simulink model "eVTOL_Small_nonandlin_algorithm_validation"  (R2024b)
settings: Solver=ode3  StartTime=0.0  StopTime=220  FixedStep=0.02  RelTol=1e-3
undefined symbols (not defined in the file): a_, b, c, c1_, deg, dttrim0, F, g, g1, h1, l1, m, MIL, PARAR, rad, rho, s, T, u_dim, ut, x_dim, xf, xmset, y_dim, yf, ymset, zf, zmset
libraries: simulink x34, aerolibconvert2 x5, aerolibwind2 x2, shared6dof x1
(part 1 of 7)
settings Model: Creator=Septemnicole  LastModifiedBy=23299
settings SolverCC: AlgebraicLoopSolver=TrustRegion
settings DataIOCC: SaveFormat=StructureWithTime  InspectSignalLogs=on  ReturnWorkspaceOutputs=off
settings OptimizationCC: LifeSpan=inf
settings DebuggingCC: UnconnectedInputMsg=warning  UnconnectedOutputMsg=warning  UnconnectedLineMsg=warning  SFExecutionAtInitializationDiag=none  UnderSpecifiedDimensionMsg=warning  ArithmeticOperatorsInVariantConditions=warning
settings HardwareCC: ProdBitPerSizeT=32  ProdBitPerPtrDiffT=32  ProdWordSize=32  ProdHWDeviceType=Specified
settings ModelReferenceCC: EnableRefExpFcnMdlSchedulingChecks=on
settings SFSimCC: SimUseLocalCustomCode=off  CustomCodeUndefinedFunction=UseInterfaceOnly
settings RTWCC: RTWUseLocalCustomCode=off  GPUComputeCapability=3.5
settings CodeAppCC: StateflowObjectComments=on

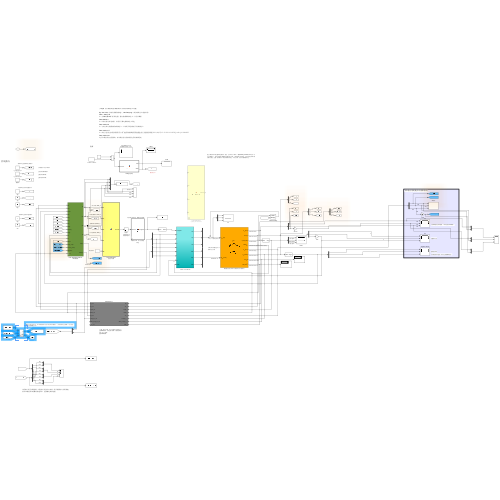
[thumbnail: Simulink's stored preview of the top-level diagram]
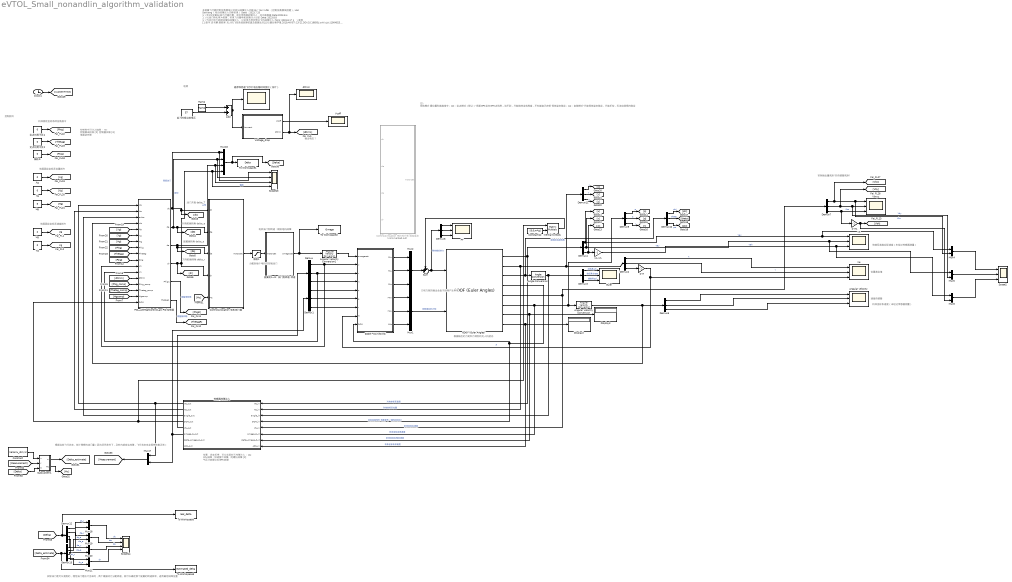
== system eVTOL_Small_nonandlin_algorithm_validation ==
  note: 实际油门是可以测到的，理性油门是估计出来的，两个根据动力分配转速，就可以确定那个旋翼的转速异常，进而确定故障位置
  note: 根据当前飞行状态，估计理想的油门量（因为闭环条件下，及时内部发生故障，飞行状态也会很快恢复正常）
  note: 方向舵偏转角 delta_r
  note: 副翼偏转角 delta_a
  note: 升降舵偏转角 delta_e
  note: 油门开度 delta_T
  note: 电机油门到转速：模拟电机故障
  note: 机体固定坐标系欧拉角指令
  note: 实际输出量观测(非传感器观测)
  note: 位置、姿态反馈，可以实现如下故障注入：
      | [1] IMU故障：加速度计故障、陀螺仪故障
      | [2] 气压计故障
      | [3] GPS故障
  note: 输出电压？
  note: 分配到每个电机的控制油门
  note: 多旋翼飞行器控制仿真模块以及部分故障注入功能
      |
      | By: Yan Xufei（控制仿真模块搭建）, Han Danyang（部分故障注入功能实现）
      | Date：2023.7.20
      | 1）完成8旋翼16轴飞行器位置、姿态传感器故障注入，并记录数据
      |
      | Date:2023.8.4
      | 1）以油门转化率为依据，实现飞行器电机故障注入设定
      |
      | Date: 2023.8.8
      | 1）气动力和力矩模块增加故障注入，以实现不受控情况下的故障注入
      |
      | Date: 2023.8.17
      | 1）参考 [1]彭宇,史书慧,郭凯等.无人机飞控系统故障仿真及数据生成[J].仪器仪表学报,2019,40(07):13-21.DOI:10.19650/j.cnki.cjsi.J1904825.
      |
      | Date: 2023.9.21
      | 1) 引入线性状态方程模块，对比线性化与复杂模型之间的相似程度
  note: 控制指令可注入故障：
      |
      | [1] 控制器未校准
      |
      | [2] 控制器失联
      |
      | [3] 地面站失联
  note: [1]: 导航模式-跟位置和速度指令；[2]：定点模式（默认）-根据GPS定在GPS点和高度（气压计+RTK）；[3]:定高模式-GPS水平模式读不到，只能维持当前高度，不知道自己在哪-保持姿态稳定；[4]：自稳模式-只能保持姿态稳定，只能手控，无法自我保持稳定
  note: 力和力矩的输出会由于故障产生异常
  note: 地轴系速度实际速度（未经过传感器测量）
  note: 根据输出的力矩和力得到的无人机姿态
  note: 电源
  note: 控制指令
  note: 位置真实值
  note: 速度传感器
  note: 地面固定坐标系位置指令
  note: 地面固定坐标系速度指令
  note: 机体坐标系速度（未经过传感器测量）
  " Angular velocity" : Scope  NumInputPorts=3
  6DOF (Euler Angles) : shared6dof/6DOF (Euler Angles)  units=Metric (MKS)  mtype=Fixed  rep=Euler Angles  xme_0=[0 0 0]  Vm_0=[0 0 0]  eul_0=[0/57.3 0/57.3 0/57.3]  pm_0=[0 0 0]  mass_0=Mass  mass_e=0.5  mass_f=2.0  inertia=Inertia  inertia_e=eye(3)  inertia_f=2*eye(3)  k_quat=1.0  vre_flag=on  abi_flag=off  aMode=aMode  xme_statename=''  Vm_statename=''  eul_statename=''  quat_statename=''  pm_statename=''  mass_statename=''
  Add : Sum
  Angle Conversion : aerolibconvert2/Angle Conversion  IU=rad  OU=deg
  Angular Velocity Conversion : aerolibconvert2/Angular Velocity Conversion  IU=rad/s  OU=deg/s
  Angular Velocity Conversion1 : aerolibconvert2/Angular Velocity Conversion  IU=rpm  OU=rad/s
  Clock1 : Clock
  Constant : Constant  Value=zeros(u_dim,1)
  Constant12 : Constant  Value=[0,0,m*g]
  ControlAllocation 电机执行器 : MATLAB Function  TreatAsAtomicUnit=on
  ControlAllocation 电机执行器-原始版本 : MATLAB Function  Commented=on  TreatAsAtomicUnit=on
  Demux{,1..7,9..11} (11 alike) : Demux  Outputs=3
  Demux12 : Demux
  Demux13 : Demux
  Display2 : Display
  Display3 : Display
  Euler : Scope  NumInputPorts=3
  FT : Scope  NumInputPorts=3
  Hg : Constant  Value=5
  Inertial to Body : Product  Multiplication=Matrix(*)  InputSameDT=on  SaturateOnIntegerOverflow=on  OutDataTypeStr=Inherit: Same as first input
  Mux1 : Mux  Inputs=3
  Mux16 : Mux
  Mux{4..6,17..21} (8 alike) : Mux  Inputs=2
  Mux2 : Mux  Inputs=3
  PID—AttHighControlLaw PID控制器 : Subsystem  mask{Ea=1}
      mask prompts: Ea "Euler angle control enable(1=disable, 2=enable)"
  Ramp : simulink/Sources/Ramp  slope=-0.05  start=0  InitialOutput=0
  Scope13 : Scope  NumInputPorts=4
  Scope14 : Scope  NumInputPorts=4
  Scope2 : Scope  NumInputPorts=3
  Subsystem1 : Subsystem
  Sum : Sum  Inputs=++|
  To Workspace : ToWorkspace  VariableName=real_delta  SaveFormat=Timeseries  SampleTime=-1
  To Workspace1 : ToWorkspace  VariableName=Delta  SaveFormat=Timeseries  SampleTime=-1
  To Workspace2 : ToWorkspace  VariableName=Omega  SaveFormat=Timeseries  SampleTime=-1
  To Workspace3 : ToWorkspace  VariableName=estimated_delta  SaveFormat=Timeseries  SampleTime=-1
  Ug : Constant  Value=2
  Vbxyz : Scope  NumInputPorts=3
  Vcoff : Scope
  Ve : Scope  NumInputPorts=3
  Vg : Constant  Value=0
  Voltage_drop : MATLAB Function  TreatAsAtomicUnit=on
  Vz-Vh : Gain  Gain=-1
  Xe : Scope  NumInputPorts=3
  Xg : Constant  Value=0
  Yg : Constant  Value=0
  Z-H : Gain  Gain=-1
  Z-H1 : Gain  Gain=-1
  dttrim : Scope
  传感器故障注入 : Subsystem  mask{Pmn=0}
      mask prompts: Pmn "the power of meansurement noise (E[S_xx]=(theta^2)/2F)"
  偏航G : Constant  Value=0
  各部件气动力和力矩 : Subsystem
  定点时用不到1 : Constant  Value=0
  定点时用不到2 : Constant  Value=0
  悬停和低速飞行时 电压随时间变化（估计） : Scope
  旋翼组1~8：油门到转速 转速 : MATLAB Function  TreatAsAtomicUnit=on  mask{L_r=1}
      mask prompts: L_r "Power loss rate from motor to omega"
  起飞时候当前电压 : Constant  Value=57
  限幅1 : Saturate  UpperLimit=1  LowerLimit=0.1
  tag scope: Ug=global, Vg=global
  wires:
  Inertial to Body/1 -> Sum/1
  6DOF (Euler Angles)/7 -> 传感器故障注入/7(delta_omega_b_in), Display3/1  "机体坐标系角加速度"
  Constant12/1 -> Inertial to Body/2
  Demux1/2 -> 各部件气动力和力矩/6(q)
  Demux1/1 -> 各部件气动力和力矩/5(p)
  Demux1/3 -> 各部件气动力和力矩/7(r)
  6DOF (Euler Angles)/8 -> 传感器故障注入/8(Abb_in), Display2/1  "机体坐标系加速度"
  6DOF (Euler Angles)/6 -> Demux9/1, Angular Velocity Conversion/1, 传感器故障注入/6(omega_b_in)  "机体坐标系角速度"
  Mux2/1 -> Sum/2
  6DOF (Euler Angles)/3 -> Demux10/1, Angle Conversion/1  "固有欧拉旋转角"
  Demux/3 -> 各部件气动力和力矩/4(w)
  [Thetag] -> PID—AttHighControlLaw PID控制器/9(Thetag)
  [Phig] -> PID—AttHighControlLaw PID控制器/8(Phig)
  Demux2/2 -> Xe/2  "Y"
  Demux2/1 -> Xe/1  "X"
  Demux2/3 -> Z-H/1
  Demux3/1 -> Euler/1  "滚转角phi"
  Demux3/2 -> Euler/2  "俯仰角theta"
  Demux3/3 -> Euler/3  "偏航角psi"
  Demux4/1 -> [u], Ve/1, Mux4/1  "Vex"
  Demux4/2 -> [v], Mux5/1, Ve/2  "Vey"
  Demux4/3 -> [w], Vz-Vh/1
  Demux5/2 -> " Angular velocity"/2
  Demux5/1 -> " Angular velocity"/1
  Demux5/3 -> " Angular velocity"/3
  Add/1 -> 悬停和低速飞行时 电压随时间变化（估计）/1, Voltage_drop/1(Vcurrent)
  起飞时候当前电压/1 -> Add/2
  Voltage_drop/2(dttrim) -> [dttrim], dttrim/1
  Voltage_drop/1(Vcoff) -> Vcoff/1
  Ramp/1 -> Add/1
  Demux6/3 -> FT/3
  Demux6/2 -> FT/2
  Demux6/1 -> FT/1
  Mux1/1 -> 6DOF (Euler Angles)/2  "刚体施加的力矩"
  Sum/1 -> 6DOF (Euler Angles)/1, Demux6/1  "刚体施加的力"
  各部件气动力和力矩/1(FAx) -> Mux2/1
  各部件气动力和力矩/2(FAy) -> Mux2/2
  各部件气动力和力矩/3(FAz) -> Mux2/3
  各部件气动力和力矩/4(MAx) -> Mux1/1
  各部件气动力和力矩/5(MAy) -> Mux1/2
  各部件气动力和力矩/6(MAz) -> Mux1/3
  Vz-Vh/1 -> Mux6/1, Ve/3  "Veh"
  [dttrim] -> PID—AttHighControlLaw PID控制器/13(dttrim)
  Angular Velocity Conversion1/1 -> 各部件气动力和力矩/1(omegaset)
  ControlAllocation 电机执行器/1(motorset) -> 限幅1/1
  Demux/2 -> 各部件气动力和力矩/3(v), PID—AttHighControlLaw PID控制器/12(v1)
  Demux/1 -> PID—AttHighControlLaw PID控制器/11(u1), 各部件气动力和力矩/2(u)
  Z-H/1 -> 各部件气动力和力矩/8(H), Xe/3  "H"
  [Xg] -> PID—AttHighControlLaw PID控制器/5(Xg)
  [Yg] -> PID—AttHighControlLaw PID控制器/6(Yg)
  Angular Velocity Conversion/1 -> Demux5/1, PID—AttHighControlLaw PID控制器/4(wb)
  Demux7/1 -> [Vbx], Mux4/2, Vbxyz/1  "Vbx"
  Demux7/2 -> Mux5/2, Vbxyz/2, [Vby]  "Vby"
  6DOF (Euler Angles)/5 -> Demux7/1, 传感器故障注入/5(Vb_in)  "机体坐标系速度"
  PID—AttHighControlLaw PID控制器/5(Phig1) -> [PhigR]  "期望滚转角"
  PID—AttHighControlLaw PID控制器/6(thetag1) -> [ThetagR]  "期望俯仰角"
  [Hg] -> PID—AttHighControlLaw PID控制器/7(Hg)
  [Phig_comp] -> PID—AttHighControlLaw PID控制器/14(Phig_comp)
  [Thetag_comp] -> PID—AttHighControlLaw PID控制器/15(Thetag_comp)
  偏航G/1 -> [Psig]
  [Psig] -> PID—AttHighControlLaw PID控制器/10(Psig)
  Xg/1 -> [Xg]
  Hg/1 -> [Hg]
  定点时用不到1/1 -> [Phig]
  定点时用不到2/1 -> [Thetag]
  [Hgcomp] -> PID—AttHighControlLaw PID控制器/16(Hgcomp)
  Z-H1/1 -> Mux6/2, [Vbh]
  Demux7/3 -> Z-H1/1, Vbxyz/3  "Vbz"
  限幅1/1 -> 旋翼组1~8：油门到转速 转速/1(motorset)
  PID—AttHighControlLaw PID控制器/1(dt) -> Scope13/1, Mux16/1, [dt], ControlAllocation 电机执行器/1(dt)  "高度油门"
  PID—AttHighControlLaw PID控制器/2(de) -> [de], ControlAllocation 电机执行器/2(de), Scope13/2, Mux16/2  "俯仰"
  PID—AttHighControlLaw PID控制器/3(da) -> ControlAllocation 电机执行器/3(da), [da], Scope13/3, Mux16/3  "滚转"
  PID—AttHighControlLaw PID控制器/4(dr) -> [dr], ControlAllocation 电机执行器/4(dr), Scope13/4, Mux16/4  "偏航"
  6DOF (Euler Angles)/1 -> Demux4/1, 传感器故障注入/1(Ve_in)  "对地坐标系速度"
  传感器故障注入/1(Ve_out) -> Mux17/1, PID—AttHighControlLaw PID控制器/1(Ve)
  传感器故障注入/2(Xe_out) -> PID—AttHighControlLaw PID控制器/2(Xe)
  6DOF (Euler Angles)/2 -> Demux2/1, Demux11/1, 传感器故障注入/2(Xe_in)  "对地坐标系位置"
  Angle Conversion/1 -> 传感器故障注入/3(angle_in), Demux3/1
  传感器故障注入/3(angle_out) -> PID—AttHighControlLaw PID控制器/3(euler)
  6DOF (Euler Angles)/4 -> 传感器故障注入/4(DCM_in), 各部件气动力和力矩/9(DCM)  "坐标变换矩阵(地面参考->固有坐标系)"
  传感器故障注入/5(Vb_out) -> Demux/1
  传感器故障注入/6(omega_b_out) -> Demux1/1, Mux17/2
  传感器故障注入/4(DCM_out) -> Inertial to Body/1, PID—AttHighControlLaw PID控制器/17(DCM)
  Yg/1 -> [Yg]
  Vg/1 -> [Vg]
  Ug/1 -> [Ug]
  旋翼组1~8：油门到转速 转速/1(omegaset) -> Angular Velocity Conversion1/1, To Workspace2/1
  Mux4/1 -> Scope2/1
  Mux5/1 -> Scope2/2
  Mux6/1 -> Scope2/3
  Demux9/1 -> [p]  "p"
  Demux9/2 -> [q]  "q"
  Demux9/3 -> [r]  "r"
  Demux10/1 -> [phi]  "phi"
  Demux10/2 -> [theta]  "theta"
  Demux10/3 -> [psi]  "psi"
  Demux11/1 -> [x]  "x"
  Demux11/2 -> [y]  "y"
  Demux11/3 -> [z]  "z"
  Clock1/1 -> [systemTime]
  Mux16/1 -> [Delta], To Workspace1/1
  [Mc] -> ControlAllocation 电机执行器/5(Mc)
  Mux17/1 -> [Measurement]
  [Measurement] -> Subsystem1/2(y)
  Subsystem1/1(w) -> [Delta_estimate]
  Subsystem1/2(Mc) -> [Mc]
  [Delta_estimate] -> To Workspace3/1, Demux13/1
  [Delta] -> To Workspace/1, Demux12/1
  Demux12/1 -> Mux18/1  "dt_r"
  Demux13/1 -> Mux18/2  "dt_e"
  Demux12/2 -> Mux19/1  "de_r"
  Demux13/2 -> Mux19/2  "de_e"
  Demux12/3 -> Mux20/1  "da_r"
  Demux13/3 -> Mux20/2  "da_e"
  Demux12/4 -> Mux21/1  "dr_r"
  Demux13/4 -> Mux21/2  "dr_e"
  Mux18/1 -> Scope14/1  "dt"
  Mux19/1 -> Scope14/2  "de"
  Mux20/1 -> Scope14/3  "da"
  Mux21/1 -> Scope14/4  "dr"
  [Delta] -> Subsystem1/3(ww)
  Constant/1 -> Subsystem1/1(u)

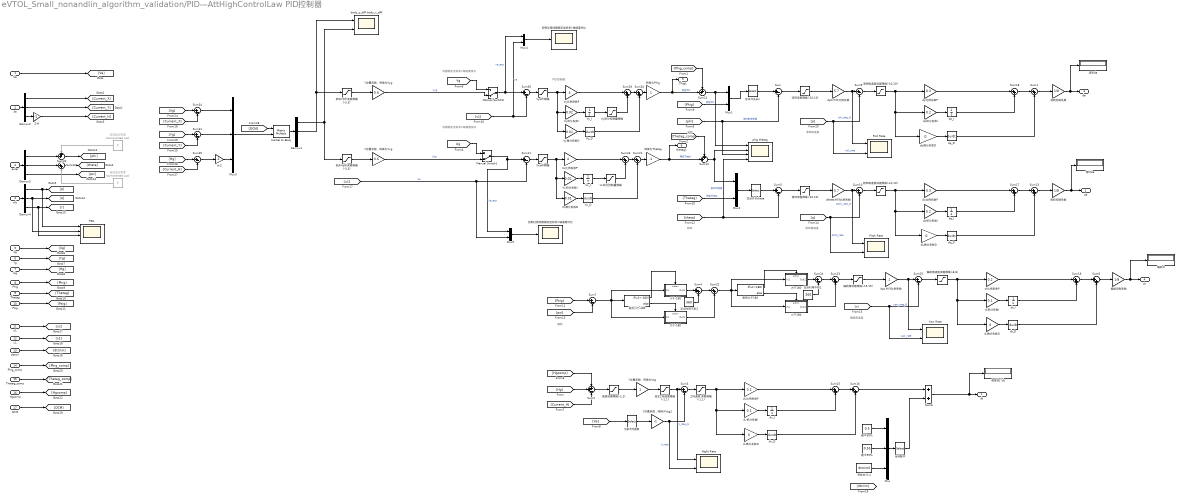
== system eVTOL_Small_nonandlin_algorithm_validation/PID—AttHighControlLaw PID控制器 ==
  note: 地面固定坐标系X轴速度指令
  note: 地面固定坐标系Y轴速度指令
  note: PID控制器
  note: 偏航
  note: 滚转角速度
  note: 俯仰角速度
  note: 俯仰
  note: 滚转
  note: 偏航角速度
  Ve : Inport
  Xe : Inport  Port=2
  euler : Inport  Port=3
  wb : Inport  Port=4
  Xg : Inport  Port=5
  Yg : Inport  Port=6
  Hg : Inport  Port=7
  Phig : Inport  Port=8
  Thetag : Inport  Port=9
  Psig : Inport  Port=10
  u1 : Inport  Port=11
  v1 : Inport  Port=12
  dttrim : Inport  Port=13
  Phig_comp : Inport  Port=14
  Thetag_comp : Inport  Port=15
  Hgcomp : Inport  Port=16
  DCM : Inport  Port=17
  Demux{1..4} (4 alike) : Demux  Outputs=3
  H-Z : Gain  Gain=-1
  Hight Rate : Scope  NumInputPorts=2
  Inertial to Body : Product  Multiplication=Matrix(*)  InputSameDT=on  SaturateOnIntegerOverflow=on  OutDataTypeStr=Inherit: Same as first input
  Manual Switch1 : ManualSwitch  CurrentSetting=0
  Manual Switch8 : ManualSwitch  CurrentSetting=0
  Mux : Mux  Inputs=3
  Mux{1..2,4..5} (4 alike) : Mux  Inputs=2
  Mux3 : Mux  Inputs=3
  PSI1 : Scope  NumInputPorts=4
  Pitch Rate : Scope  NumInputPorts=2
  Roll Rate : Scope  NumInputPorts=2
  Sum{,3,5,7,9..11,24..25,30..31,34..35} (13 alike) : Sum  Inputs=|+-
  Sum{1,4,8,13,15..23,26,29,33} (16 alike) : Sum  Inputs=|++
  Sum12 : Sum  Inputs=++|
  Sum14 : Sum  Inputs=++|
  Sum2 : Sum  Inputs=++-
  Sum32 : Sum  Inputs=++|
  Sum6 : Sum
  Vx_D : Derivative
  Vx_I : Integrator
  Vxdiff限幅 : Saturate  UpperLimit=2.4  LowerLimit=-2.4
  Vx微分系数D : Gain  Gain=0.01
  Vx比例系数P : Gain  Gain=4
  Vx积分控制量限幅 : Saturate  UpperLimit=2  LowerLimit=-2
  Vx积分系数I : Gain  Gain=0.02
  Vy_D : Derivative
  Vy_I : Integrator
  Vydiff限幅 : Saturate  UpperLimit=2.4  LowerLimit=-2.4
  Vy微分系数D : Gain  Gain=0.01
  Vy比例系数P : Gain  Gain=4
  Vy积分控制量限幅 : Saturate  UpperLimit=2  LowerLimit=-2
  Vy积分系数I : Gain  Gain=0.02
  X位置系数，转换为Vxg : Gain  Gain=0.6
  Yaw Rate : Scope  NumInputPorts=2
  Y位置系数，转换为Vyg : Gain  Gain=0.6
  Y位置系数，转换为Vzg : Gain
  Y位置系数，转换为Vzg1 : Gain  Gain=-1
  Z-H : Gain  Gain=-1
  Z向速度 误差限幅 (-1,1) : Saturate  UpperLimit=1  LowerLimit=-1
  body_y_diff body_x_diff : Scope  NumInputPorts=2
  dp_D : Derivative
  dp_I : Integrator
  dphi外环比例系数 : Gain  Gain=5.7
  dpsi外环比例系数 : Gain
  dp微分系数D : Gain  Gain=0
  dp比例系数P : Gain  Gain=0.3
  dp积分系数I : Gain  Gain=0.2
  dq_D : Derivative
  dq_I : Integrator
  dq微分系数D : Gain  Gain=0
  dq比例系数P : Gain  Gain=0.3
  dq积分系数I : Gain  Gain=0.2
  dr_D : Derivative
  dr_I : Integrator
  dr微分系数D : Gain  Gain=0
  dr比例系数P : Gain  Gain=0.2
  dr积分系数I : Gain  Gain=0.1
  dtheta外环比例系数 : Gain  Gain=5.7
  dv_D : Derivative
  dv_I : Integrator
  dv微分系数D : Gain  Gain=0
  dv比例系数P : Gain  Gain=0.2
  dv积分系数I : Gain  Gain=0.1
  phig thetag : Scope  NumInputPorts=4
  俯仰de : Display
  俯仰姿态零漂 : Constant  Commented=on  Value=0
  俯仰控制系数 : Gain  Gain=1/8
  俯仰角速度误差限幅(-10,10) : Saturate  UpperLimit=10  LowerLimit=-10
  "俯仰误差限幅(-10,10) " : Saturate  UpperLimit=10  LowerLimit=-10
  偏航dr : Display
  偏航控制系数 : Gain  Gain=1/8
  "偏航角误差限幅(-15,15) " : Saturate  UpperLimit=15  LowerLimit=-15
  偏航角速度误差限幅(-8,8) : Saturate  UpperLimit=8  LowerLimit=-8
  "初始dt 0.4 " : Constant  Value=dttrim0
  大于-180 : Subsystem  TreatAsAtomicUnit=on
  大于180 : Subsystem  TreatAsAtomicUnit=on
  定点开关phi : Selector  InputPortWidth=2  IndexOptions=Index vector (dialog)  Indices=[Ea]  OutputSizes=1
  定点开关theta : Selector  InputPortWidth=2  IndexOptions=Index vector (dialog)  Indices=[Ea]  OutputSizes=1
  定点时用不到1 : Constant  Value=360
  定点时用不到2 : Constant  Value=360
  小于-180 : Subsystem  TreatAsAtomicUnit=on
  小于180 : Subsystem  TreatAsAtomicUnit=on
  当前Z向速度 : Selector  InputPortWidth=3  IndexOptions=Index vector (dialog)  Indices=[3]  OutputSizes=1
  当前配平 : Selector  InputPortWidth=3  IndexOptions=Index vector (dialog)  Indices=[3]  OutputSizes=1
  控制过程地面固定坐标系X轴速度对比 : Scope
  控制过程地面固定坐标系Y轴速度对比 : Scope
  是否大于180 : If  IfExpression=u1>180
  是否小于-180 : If  IfExpression=u1<-180
  机体Xdiff误差限幅 (-3,3) : Saturate  UpperLimit=3  LowerLimit=-3
  机体Ydiff误差限幅 (-3,3) : Saturate  UpperLimit=3  LowerLimit=-3
  滚转da : Display
  滚转姿态零漂 : Constant  Commented=on  Value=0
  滚转控制系数 : Gain  Gain=1/8
  滚转角速度误差限幅(-10,10) : Saturate  UpperLimit=10  LowerLimit=-10
  "滚转误差限幅(-10,10) " : Saturate  UpperLimit=10  LowerLimit=-10
  给定Z向速度限幅 (-1,1) : Saturate  UpperLimit=1  LowerLimit=-1
  转换为Phig : Gain
  转换为Thetag : Gain  Gain=-1
  "配平50% " : Constant  Value=0.5
  配平55% : Constant  Value=0.55
  高度油门dt : Display
  高度误差限幅(-2,2) : Saturate  UpperLimit=2  LowerLimit=-2
  dt : Outport  VectorParamsAs1DForOutWhenUnconnected=off
  de : Outport  Port=2  VectorParamsAs1DForOutWhenUnconnected=off
  da : Outport  Port=3  VectorParamsAs1DForOutWhenUnconnected=off
  dr : Outport  Port=4  VectorParamsAs1DForOutWhenUnconnected=off
  Phig1 : Outport  Port=5  VectorParamsAs1DForOutWhenUnconnected=off
  thetag1 : Outport  Port=6  VectorParamsAs1DForOutWhenUnconnected=off
  wires:
  euler/1 -> Demux3/1
  Demux4/1 -> PSI1/1, [p]
  Demux4/2 -> PSI1/2, [q]
  Thetag/1 -> [Thetag]
  wb/1 -> Demux4/1
  Hg/1 -> [Hg]
  Demux4/3 -> PSI1/3, [r]
  Yg/1 -> [Yg]
  Demux3/3 -> [psi]
  Demux2/3 -> Z-H/1
  Xe/1 -> Demux2/1
  Psig/1 -> [Psig]
  u1/1 -> [u1]
  v1/1 -> [v1]
  dttrim/1 -> [dttrim]
  Sum32/1 -> [phi]
  Demux3/1 -> Sum32/2
  滚转姿态零漂/1 -> Sum32/1
  Sum33/1 -> [theta]
  Demux3/2 -> Sum33/1
  俯仰姿态零漂/1 -> Sum33/2
  Demux2/1 -> [Current_X]
  Demux2/2 -> [Current_Y]
  Z-H/1 -> [Current_H]
  Xg/1 -> [Xg]
  Phig/1 -> [Phig]
  Sum22/1 -> 大于180/1(In1), 小于180/1(In1), 是否大于180/1
  Sum16/1 -> Sum6/1
  Mux2/1 -> 定点开关theta/1
  Sum18/1 -> Sum1/1
  dtheta外环比例系数/1 -> Pitch Rate/1, Sum10/1  "pitch_rate_G"
  Vy积分系数I/1 -> Vy_I/1
  配平55%/1 -> Mux/2
  Y位置系数，转换为Vzg1/1 -> Hight Rate/2, Sum3/2  "h_rate"
  是否小于-180/1 -> 小于-180/Action
  [p] -> Roll Rate/2, Sum9/2  "roll_rate"
  dq积分系数I/1 -> dq_I/1
  Sum20/1 -> 转换为Phig/1
  dp_D/1 -> Sum1/2
  [v1] -> Mux4/2, Sum30/2  "Ve"
  Y位置系数，转换为Vyg/1 -> Manual Switch8/2  "Vyg"
  Vx_I/1 -> Vx积分控制量限幅/1
  Sum21/1 -> 转换为Thetag/1
  dphi外环比例系数/1 -> Roll Rate/1, Sum9/1  "roll_rate_G"
  dq_D/1 -> Sum13/2
  Vx积分系数I/1 -> Vx_I/1
  Sum15/1 -> Sum16/1
  dp_I/1 -> Sum18/2
  dv_I/1 -> Sum15/2
  俯仰角速度误差限幅(-10,10)/1 -> dq微分系数D/1, dq积分系数I/1, dq比例系数P/1
  dq比例系数P/1 -> Sum17/1
  [Ve] -> 当前Z向速度/1
  [theta] -> Sum5/2, phig thetag/4  "俯仰传感器"
  Vy微分系数D/1 -> Vy_D/1
  Vy积分控制量限幅/1 -> Sum29/2
  Vy_I/1 -> Vy积分控制量限幅/1
  俯仰控制系数/1 -> 俯仰de/1, de/1
  "偏航角误差限幅(-15,15) "/1 -> dpsi外环比例系数/1
  Vydiff限幅/1 -> Vy微分系数D/1, Vy积分系数I/1, Vy比例系数P/1
  Sum8/1 -> 偏航控制系数/1
  机体Ydiff误差限幅 (-3,3)/1 -> Y位置系数，转换为Vyg/1
  Vxdiff限幅/1 -> Vx微分系数D/1, Vx积分系数I/1, Vx比例系数P/1
  大于180/1(Out1) -> Sum24/1
  Vx比例系数P/1 -> Sum26/1
  dr_I/1 -> Sum19/2
  Mux1/1 -> 定点开关phi/1
  给定Z向速度限幅 (-1,1)/1 -> Hight Rate/1, Sum3/1  "h_rate_G"
  转换为Thetag/1 -> Sum14/2, thetag1/1  "期望Theta"
  滚转控制系数/1 -> 滚转da/1, da/1
  转换为Phig/1 -> Phig1/1, Sum12/2  "期望Phi"
  dv_D/1 -> Sum16/2
  [q] -> Pitch Rate/2, Sum10/2  "pitch_rate"
  Vy_D/1 -> Sum20/2
  dv微分系数D/1 -> dv_D/1
  dv积分系数I/1 -> dv_I/1
  dr积分系数I/1 -> dr_I/1
  dq微分系数D/1 -> dq_D/1
  Sum13/1 -> 俯仰控制系数/1
  [Psig] -> Sum7/1
  dr微分系数D/1 -> dr_D/1
  偏航角速度误差限幅(-8,8)/1 -> dr微分系数D/1, dr积分系数I/1, dr比例系数P/1
  dq_I/1 -> Sum17/2
  dv比例系数P/1 -> Sum15/1
  Sum17/1 -> Sum13/1
  Sum19/1 -> Sum8/1
  dp积分系数I/1 -> dp_I/1
  偏航控制系数/1 -> 偏航dr/1, dr/1
  Y位置系数，转换为Vzg/1 -> 给定Z向速度限幅 (-1,1)/1
  [psi] -> Sum7/2
  Vx微分系数D/1 -> Vx_D/1
  Sum10/1 -> 俯仰角速度误差限幅(-10,10)/1
  Sum30/1 -> Vydiff限幅/1
  [phi] -> phig thetag/3, Sum/2  "滚转角传感器"
  定点开关phi/1 -> Sum/1
  Vy比例系数P/1 -> Sum29/1
  Vx积分控制量限幅/1 -> Sum26/2
  "初始dt 0.4 "/1 -> Mux/3
  X位置系数，转换为Vxg/1 -> Manual Switch1/2  "Uxg"
  定点时用不到1/1 -> Sum24/2
  [Thetag] -> Mux2/2  "期望Theta"
  机体Xdiff误差限幅 (-3,3)/1 -> X位置系数，转换为Vxg/1
  Sum5/1 -> "俯仰误差限幅(-10,10) "/1
  是否小于-180/2 -> 大于-180/Action
  高度误差限幅(-2,2)/1 -> Y位置系数，转换为Vzg/1
  dpsi外环比例系数/1 -> Yaw Rate/1, Sum25/1  "yaw_rate_G"
  Z向速度 误差限幅 (-1,1)/1 -> dv微分系数D/1, dv积分系数I/1, dv比例系数P/1
  Sum7/1 -> 大于-180/1(In1), 小于-180/1(In1), 是否小于-180/1
  Sum3/1 -> Z向速度 误差限幅 (-1,1)/1
  dp微分系数D/1 -> dp_D/1
  是否大于180/2 -> 小于180/Action
  是否大于180/1 -> 大于180/Action
  dr比例系数P/1 -> Sum19/1
  Mux/1 -> 当前配平/1
  Sum23/1 -> "偏航角误差限幅(-15,15) "/1
  定点开关theta/1 -> Sum5/1
  Sum2/1 -> 高度误差限幅(-2,2)/1
  Sum25/1 -> 偏航角速度误差限幅(-8,8)/1
  [r] -> Yaw Rate/2, Sum25/2  "yaw_rate"
  当前配平/1 -> Sum6/2
  "滚转误差限幅(-10,10) "/1 -> dphi外环比例系数/1
  Sum24/1 -> Sum23/1
  dp比例系数P/1 -> Sum18/1
  Sum4/1 -> Sum22/1
  小于180/1(Out1) -> Sum23/2
  "俯仰误差限幅(-10,10) "/1 -> dtheta外环比例系数/1
  Sum11/1 -> Vxdiff限幅/1
  Sum6/1 -> 高度油门dt/1, dt/1
  定点时用不到2/1 -> Sum4/2
  [Phig] -> Mux1/2  "期望Phi"
  Sum9/1 -> 滚转角速度误差限幅(-10,10)/1
  "配平50% "/1 -> Mux/1
  当前Z向速度/1 -> Y位置系数，转换为Vzg1/1
  滚转角速度误差限幅(-10,10)/1 -> dp比例系数P/1, dp微分系数D/1, dp积分系数I/1
  大于-180/1(Out1) -> Sum22/2
  dr_D/1 -> Sum8/2
  Sum1/1 -> 滚转控制系数/1
  小于-180/1(Out1) -> Sum4/1
  Sum/1 -> "滚转误差限幅(-10,10) "/1
  Phig_comp/1 -> [Phig_comp]
  Thetag_comp/1 -> [Thetag_comp]
  Sum12/1 -> phig thetag/1, Mux1/1
  [Phig_comp] -> Sum12/1
  Sum29/1 -> Sum20/1
  [Thetag_comp] -> Sum14/1
  Sum26/1 -> Sum21/1
  Vx_D/1 -> Sum21/2
  Sum14/1 -> Mux2/1, phig thetag/2
  [Hg] -> Sum2/2
  [Current_H] -> Sum2/3
  Demux1/1 -> 机体Xdiff误差限幅 (-3,3)/1, body_y_diff body_x_diff/2
  Demux1/2 -> body_y_diff body_x_diff/1, 机体Ydiff误差限幅 (-3,3)/1
  Sum34/1 -> Mux3/1
  [Hg] -> Sum35/1
  Inertial to Body/1 -> Demux1/1
  Mux3/1 -> Inertial to Body/2
  [Current_X] -> Sum34/2
  [Xg] -> Sum34/1
  [Current_Y] -> Sum31/2
  [Yg] -> Sum31/1
  H-Z/1 -> Mux3/3
  [Current_H] -> Sum35/2
  Sum35/1 -> H-Z/1
  Sum31/1 -> Mux3/2
  [DCM] -> Inertial to Body/1
  DCM/1 -> [DCM]
  Hgcomp/1 -> [Hgcomp]
  [Hgcomp] -> Sum2/1
  Ve/1 -> [Ve]
  [Vg] -> Manual Switch8/1
  [Ug] -> Manual Switch1/1
  Manual Switch8/1 -> Mux4/1, Sum30/1  "Ve_exp"
  Mux4/1 -> 控制过程地面固定坐标系Y轴速度对比/1
  [u1] -> Mux5/2, Sum11/2  "Ve"
  Mux5/1 -> 控制过程地面固定坐标系X轴速度对比/1
  Manual Switch1/1 -> Mux5/1, Sum11/1  "Ue_exp"

== system eVTOL_Small_nonandlin_algorithm_validation/Subsystem1 ==
  note: 实测油门总量
  note: 估计油门总量
  u : Inport
  y : Inport  Port=2
  ww : Inport  Port=3
  Clock : Clock
  MATLAB Function : MATLAB Function  TreatAsAtomicUnit=on
  MATLAB Function1 : MATLAB Function  TreatAsAtomicUnit=on
  Scope : Scope
  Subsystem1 : Subsystem
  w : Outport
  Mc : Outport  Port=2
  wires:
  y/1 -> Subsystem1/2(y)
  u/1 -> Subsystem1/1(u)
  MATLAB Function/1(Mc) -> Mc/1, Scope/1
  Subsystem1/1(w) -> w/1, MATLAB Function/2(Delta_estimate)
  Clock/1 -> MATLAB Function1/1(t), MATLAB Function/4(t)
  ww/1 -> MATLAB Function/1(Delta_measure), Subsystem1/3(ww)
  MATLAB Function1/1(P) -> MATLAB Function/3(P)

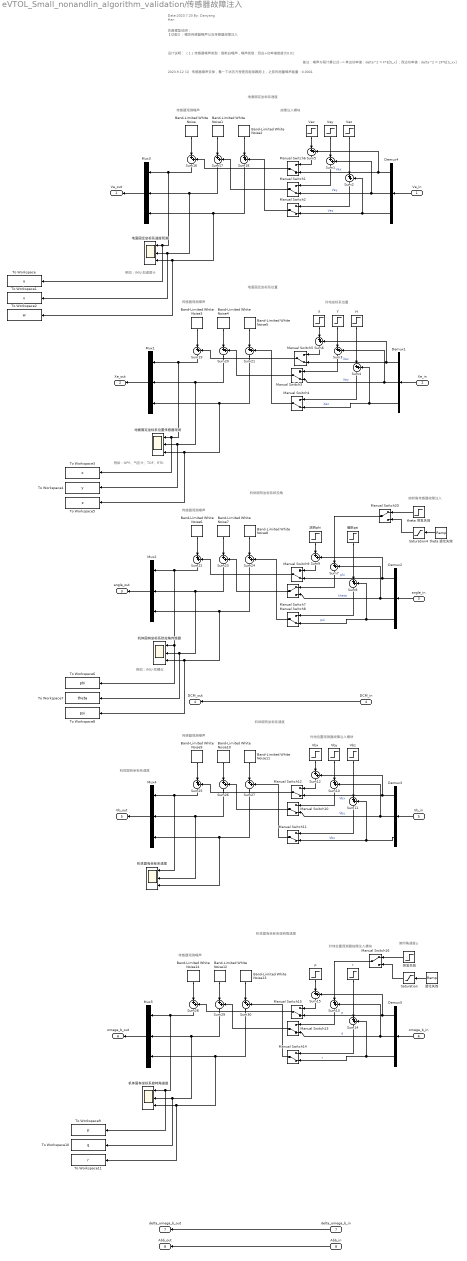
== system eVTOL_Small_nonandlin_algorithm_validation/传感器故障注入 ==
  note: 2023.9.12
      |
      | (1) 传感器噪声去掉，看一下状态方程是否能够跟踪上，之前的测量噪声能量：0.0001
  note: 俯仰角速度q
  note: 机体固有坐标系欧拉角
  note: 备注：噪声方程计算公式--> 单边功率谱：delta^2 = F*E[S_x]；双边功率谱：delta^2 = 2F*E[S_xx]
  note: 设计说明：
      |
      | （1）传感器噪声类型：高斯白噪声，噪声类型：双边+功率谱密度为0.01
  note: Date:2023.7.20
      | By: Danyang Han
  note: 仿真模型说明：
      |
      | 【功能】：模仿传感器噪声以及传感器故障注入
  note: 例如：IMU-加速度计
  note: 例如：IMU-陀螺仪
  note: 例如：GPS、气压计、TOF、RTK
  note: 传感器观测噪声
  note: 故障注入模块
  note: 对地坐标系位置
  note: 对地位置观测器故障注入模块
  note: 对地位置观测器故障注入模块
  note: 地面固定坐标系速度
  note: 传感器观测噪声
  note: 传感器观测噪声
  note: 传感器观测噪声
  note: 传感器观测噪声
  note: 地面固定坐标系位置
  note: 机体固有坐标系速度
  note: 机体固有坐标系速度
  note: 机体固有坐标系旋转角速度
  note: 俯仰角传感器故障注入
  Ve_in : Inport
  Xe_in : Inport  Port=2
  angle_in : Inport  Port=3
  DCM_in : Inport  Port=4
  Vb_in : Inport  Port=5
  omega_b_in : Inport  Port=6
  delta_omega_b_in : Inport  Port=7
  Abb_in : Inport  Port=8
  Band-Limited White Noise{,1..14} (15 alike) : simulink/Sources/Band-Limited White Noise  Cov=[Pmn]  Ts=0.1  seed=[23341]
  Demux{1..5} (5 alike) : Demux  Outputs=3
  H : Step  Time=30  After=0.5  SampleTime=0
  Manual Switch{1..6,8..15} (14 alike) : ManualSwitch  CurrentSetting=0
  Manual Switch16 : ManualSwitch
  Manual Switch20 : ManualSwitch
  Manual Switch7 : ManualSwitch
  Mux{1..5} (5 alike) : Mux  Inputs=3
  Saturation : Saturate  UpperLimit=10  LowerLimit=0
  Saturation4 : Saturate  UpperLimit=10  LowerLimit=0
  Sum{1..30} (30 alike) : Sum  Inputs=|++
  To Workspace : ToWorkspace  VariableName=u  SaveFormat=Timeseries  SampleTime=-1
  To Workspace1 : ToWorkspace  VariableName=v  SaveFormat=Timeseries  SampleTime=-1
  To Workspace10 : ToWorkspace  VariableName=q  SaveFormat=Timeseries  SampleTime=-1
  To Workspace11 : ToWorkspace  VariableName=r  SaveFormat=Timeseries  SampleTime=-1
  To Workspace2 : ToWorkspace  VariableName=w  SaveFormat=Timeseries  SampleTime=-1
  To Workspace3 : ToWorkspace  VariableName=x  SaveFormat=Timeseries  SampleTime=-1
  To Workspace4 : ToWorkspace  VariableName=y  SaveFormat=Timeseries  SampleTime=-1
  To Workspace5 : ToWorkspace  VariableName=z  SaveFormat=Timeseries  SampleTime=-1
  To Workspace6 : ToWorkspace  VariableName=phi  SaveFormat=Timeseries  SampleTime=-1
  To Workspace7 : ToWorkspace  VariableName=theta  SaveFormat=Timeseries  SampleTime=-1
  To Workspace8 : ToWorkspace  VariableName=psi  SaveFormat=Timeseries  SampleTime=-1
  To Workspace9 : ToWorkspace  VariableName=p  SaveFormat=Timeseries  SampleTime=-1
  Vbx : Step  Time=30  After=0.2  SampleTime=0
  Vby : Step  Time=30  After=0.2  SampleTime=0
  Vbz : Step  Time=30  After=0.5  SampleTime=0
  Vex : Step  Time=30  After=0.2  SampleTime=0
  Vey : Step  Time=30  After=0.2  SampleTime=0
  Vez : Step  Time=30  After=0.5  SampleTime=0
  X : Step  Time=30  After=0.2  SampleTime=0
  Y : Step  Time=30  After=0.2  SampleTime=0
  p : Step  Time=30  After=0.2  SampleTime=0
  r : Step  Time=30  After=0.5  SampleTime=0
  theta 突发失效 : Step  Time=120  After=5  SampleTime=0
  theta 退化失效 : simulink/Sources/Ramp  slope=0.3325  start=30  InitialOutput=0
  偏航psi : Step  Time=30  After=0.5  SampleTime=0
  地面固定坐标系位置传感器观测 : Scope  NumInputPorts=3
  地面固定坐标系速度观测 : Scope  NumInputPorts=3
  机体固有坐标系旋转角速度 : Scope  NumInputPorts=3
  机体固有坐标系欧拉角传感器 : Scope  NumInputPorts=3
  机体固有坐标系速度 : Scope  NumInputPorts=3
  滚转phi : Step  Time=30  After=0.2  SampleTime=0
  突发失效 : Step  Time=30  After=5  SampleTime=0
  退化失效 : simulink/Sources/Ramp  slope=0.0325  start=30  InitialOutput=0
  Ve_out : Outport
  Xe_out : Outport  Port=2
  angle_out : Outport  Port=3
  DCM_out : Outport  Port=4
  Vb_out : Outport  Port=5
  omega_b_out : Outport  Port=6
  delta_omega_b_out : Outport  Port=7
  Abb_out : Outport  Port=8
  wires:
  DCM_in/1 -> DCM_out/1
  delta_omega_b_in/1 -> delta_omega_b_out/1
  Abb_in/1 -> Abb_out/1
  Demux1/1 -> Manual Switch5/2, Sum6/2  "Xex"
  X/1 -> Sum6/1
  Xe_in/1 -> Demux1/1
  Demux1/2 -> Sum3/2, Manual Switch3/2  "Xey"
  Y/1 -> Sum3/1
  Sum3/1 -> Manual Switch3/1
  Sum6/1 -> Manual Switch5/1
  Mux1/1 -> Xe_out/1
  Demux1/3 -> Sum4/2, Manual Switch4/2  "Xez"
  Sum4/1 -> Manual Switch4/1
  H/1 -> Sum4/1
  Demux2/1 -> Manual Switch9/2, Sum9/2  "phi"
  滚转phi/1 -> Sum9/1
  Sum9/1 -> Manual Switch9/1
  Demux2/2 -> Sum7/2, Manual Switch7/2  "theta"
  Sum7/1 -> Manual Switch7/1
  angle_in/1 -> Demux2/1
  偏航psi/1 -> Sum8/1
  Sum8/1 -> Manual Switch8/1
  Demux2/3 -> Sum8/2, Manual Switch8/2  "psi"
  Mux2/1 -> angle_out/1
  Vb_in/1 -> Demux3/1
  Demux3/2 -> Sum10/2, Manual Switch10/2  "Vby"
  Demux3/3 -> Sum11/2, Manual Switch11/2  "Vbz"
  Mux4/1 -> Vb_out/1
  Demux3/1 -> Manual Switch12/2, Sum12/2  "Vbx"
  Vby/1 -> Sum10/1
  Sum12/1 -> Manual Switch12/1
  Vbz/1 -> Sum11/1
  Sum10/1 -> Manual Switch10/1
  Sum11/1 -> Manual Switch11/1
  Vbx/1 -> Sum12/1
  Demux5/3 -> Sum14/2, Manual Switch14/2  "r"
  Demux5/1 -> Manual Switch15/2, Sum15/2  "p"
  Sum15/1 -> Manual Switch15/1
  p/1 -> Sum15/1
  r/1 -> Sum14/1
  omega_b_in/1 -> Demux5/1
  Sum14/1 -> Manual Switch14/1
  Demux5/2 -> Sum13/2, Manual Switch13/2  "q"
  Mux5/1 -> omega_b_out/1
  Sum13/1 -> Manual Switch13/1
  Demux4/1 -> Manual Switch6/2, Sum5/2  "Vex"
  Vex/1 -> Sum5/1
  Sum5/1 -> Manual Switch6/1
  Demux4/2 -> Sum1/2, Manual Switch1/2  "Vey"
  Sum1/1 -> Manual Switch1/1
  Ve_in/1 -> Demux4/1
  Vey/1 -> Sum1/1
  Vez/1 -> Sum2/1
  Sum2/1 -> Manual Switch2/1
  Demux4/3 -> Sum2/2, Manual Switch2/2  "Vez"
  Mux3/1 -> Ve_out/1
  Sum16/1 -> To Workspace/1, 地面固定坐标系速度观测/1, Mux3/1
  Manual Switch6/1 -> Sum16/2
  Band-Limited White Noise/1 -> Sum16/1
  Band-Limited White Noise1/1 -> Sum17/1
  Band-Limited White Noise2/1 -> Sum18/1
  Manual Switch1/1 -> Sum17/2
  Sum17/1 -> To Workspace1/1, 地面固定坐标系速度观测/2, Mux3/2
  Manual Switch2/1 -> Sum18/2
  Sum18/1 -> To Workspace2/1, 地面固定坐标系速度观测/3, Mux3/3
  Manual Switch3/1 -> Sum20/2
  Manual Switch5/1 -> Sum19/2
  Manual Switch4/1 -> Sum21/2
  Band-Limited White Noise3/1 -> Sum19/1
  Band-Limited White Noise5/1 -> Sum21/1
  Band-Limited White Noise4/1 -> Sum20/1
  Manual Switch8/1 -> Sum24/2
  Manual Switch9/1 -> Sum22/2
  Band-Limited White Noise7/1 -> Sum23/1
  Manual Switch7/1 -> Sum23/2
  Band-Limited White Noise8/1 -> Sum24/1
  Band-Limited White Noise6/1 -> Sum22/1
  Sum27/1 -> 机体固有坐标系速度/3, Mux4/3
  Manual Switch12/1 -> Sum25/2
  Sum26/1 -> 机体固有坐标系速度/2, Mux4/2
  Band-Limited White Noise11/1 -> Sum27/1
  Band-Limited White Noise10/1 -> Sum26/1
  Band-Limited White Noise9/1 -> Sum25/1
  Sum25/1 -> 机体固有坐标系速度/1, Mux4/1
  Manual Switch11/1 -> Sum27/2
  Manual Switch10/1 -> Sum26/2
  Band-Limited White Noise14/1 -> Sum28/1
  Band-Limited White Noise13/1 -> Sum30/1
  Band-Limited White Noise12/1 -> Sum29/1
  Manual Switch14/1 -> Sum30/2
  Manual Switch13/1 -> Sum29/2
  Manual Switch15/1 -> Sum28/2
  Manual Switch16/1 -> Sum13/1
  突发失效/1 -> Manual Switch16/1
  退化失效/1 -> Saturation/1
  Saturation/1 -> Manual Switch16/2
  theta 突发失效/1 -> Manual Switch20/1
  theta 退化失效/1 -> Saturation4/1
  Saturation4/1 -> Manual Switch20/2
  Manual Switch20/1 -> Sum7/1
  Sum19/1 -> Mux1/1, To Workspace3/1, 地面固定坐标系位置传感器观测/1
  Sum20/1 -> 地面固定坐标系位置传感器观测/2, To Workspace4/1, Mux1/2
  Sum21/1 -> 地面固定坐标系位置传感器观测/3, To Workspace5/1, Mux1/3
  Sum22/1 -> 机体固有坐标系欧拉角传感器/1, To Workspace6/1, Mux2/1
  Sum24/1 -> To Workspace8/1, 机体固有坐标系欧拉角传感器/3, Mux2/3
  Sum23/1 -> To Workspace7/1, 机体固有坐标系欧拉角传感器/2, Mux2/2
  Sum30/1 -> Mux5/3, To Workspace11/1, 机体固有坐标系旋转角速度/3
  Sum29/1 -> To Workspace10/1, 机体固有坐标系旋转角速度/2, Mux5/2
  Sum28/1 -> To Workspace9/1, 机体固有坐标系旋转角速度/1, Mux5/1

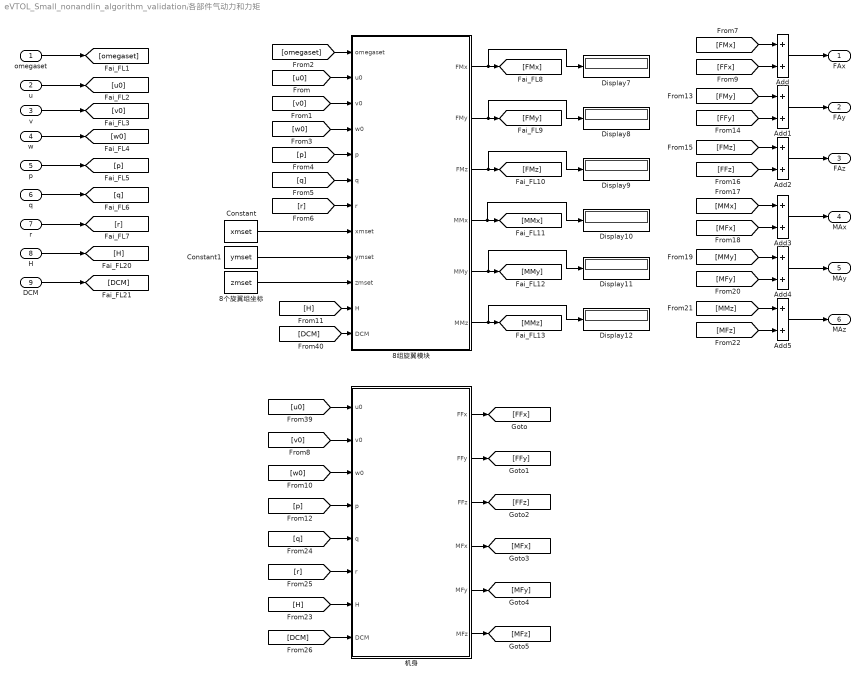
== system eVTOL_Small_nonandlin_algorithm_validation/各部件气动力和力矩 ==
  omegaset : Inport
  u : Inport  Port=2
  v : Inport  Port=3
  w : Inport  Port=4
  p : Inport  Port=5
  q : Inport  Port=6
  r : Inport  Port=7
  H : Inport  Port=8
  DCM : Inport  Port=9
  8个旋翼组坐标 : Constant  Value=zmset
  8组旋翼模块 : Subsystem  mask{Lp=0.5, Tf=220}
      mask prompts: Lp "Power loss rate on motor"; Tf "Start time of fault injection"
  Add{,1..5} (6 alike) : Sum
  Constant : Constant  Value=xmset
  Constant1 : Constant  Value=ymset
  Display{7..12} (6 alike) : Display
  机身 : Subsystem
  FAx : Outport  VectorParamsAs1DForOutWhenUnconnected=off
  FAy : Outport  Port=2  VectorParamsAs1DForOutWhenUnconnected=off
  FAz : Outport  Port=3  VectorParamsAs1DForOutWhenUnconnected=off
  MAx : Outport  Port=4  VectorParamsAs1DForOutWhenUnconnected=off
  MAy : Outport  Port=5  VectorParamsAs1DForOutWhenUnconnected=off
  MAz : Outport  Port=6  VectorParamsAs1DForOutWhenUnconnected=off
  wires:
  omegaset/1 -> [omegaset]
  [omegaset] -> 8组旋翼模块/1(omegaset)
  r/1 -> [r]
  q/1 -> [q]
  p/1 -> [p]
  [p] -> 8组旋翼模块/5(p)
  [q] -> 8组旋翼模块/6(q)
  [r] -> 8组旋翼模块/7(r)
  Constant/1 -> 8组旋翼模块/8(xmset)
  Constant1/1 -> 8组旋翼模块/9(ymset)
  8个旋翼组坐标/1 -> 8组旋翼模块/10(zmset)
  Add/1 -> FAx/1
  Add1/1 -> FAy/1
  [FMx] -> Add/1
  [FFx] -> Add/2
  [FFy] -> Add1/2
  [FMy] -> Add1/1
  [FMz] -> Add2/1
  [FFz] -> Add2/2
  Add2/1 -> FAz/1
  [MFx] -> Add3/2
  [MMx] -> Add3/1
  Add3/1 -> MAx/1
  [MMy] -> Add4/1
  [MFy] -> Add4/2
  Add4/1 -> MAy/1
  [MFz] -> Add5/2
  [MMz] -> Add5/1
  Add5/1 -> MAz/1
  8组旋翼模块/1(FMx) -> Display7/1, [FMx]
  8组旋翼模块/2(FMy) -> Display8/1, [FMy]
  8组旋翼模块/3(FMz) -> Display9/1, [FMz]
  8组旋翼模块/4(MMx) -> Display10/1, [MMx]
  8组旋翼模块/5(MMy) -> Display11/1, [MMy]
  8组旋翼模块/6(MMz) -> Display12/1, [MMz]
  u/1 -> [u0]
  v/1 -> [v0]
  w/1 -> [w0]
  [u0] -> 8组旋翼模块/2(u0)
  [v0] -> 8组旋翼模块/3(v0)
  [w0] -> 8组旋翼模块/4(w0)
  H/1 -> [H]
  DCM/1 -> [DCM]
  机身/1(FFx) -> [FFx]
  机身/2(FFy) -> [FFy]
  机身/3(FFz) -> [FFz]
  机身/4(MFx) -> [MFx]
  机身/5(MFy) -> [MFy]
  机身/6(MFz) -> [MFz]
  [u0] -> 机身/1("u0 ")
  [v0] -> 机身/2(v0)
  [w0] -> 机身/3(w0)
  [p] -> 机身/4(p)
  [q] -> 机身/5(q)
  [r] -> 机身/6(r)
  [H] -> 8组旋翼模块/11(H)
  [DCM] -> 8组旋翼模块/12(DCM)
  [H] -> 机身/7(H)
  [DCM] -> 机身/8(DCM)

== system eVTOL_Small_nonandlin_algorithm_validation/PID—AttHighControlLaw PID控制器/大于-180 ==
  In1 : Inport
  Action Port : ActionPort  ActionPortLabel=else
  Out1 : Outport  VectorParamsAs1DForOutWhenUnconnected=off
  wires:
  In1/1 -> Out1/1

== system eVTOL_Small_nonandlin_algorithm_validation/PID—AttHighControlLaw PID控制器/大于180 ==
  In1 : Inport
  Action Port : ActionPort  ActionPortLabel=if(u1>180)
  Out1 : Outport  VectorParamsAs1DForOutWhenUnconnected=off
  wires:
  In1/1 -> Out1/1

== system eVTOL_Small_nonandlin_algorithm_validation/PID—AttHighControlLaw PID控制器/小于-180 ==
  In1 : Inport
  Action Port : ActionPort  ActionPortLabel=if(u1<-180)
  Out1 : Outport  VectorParamsAs1DForOutWhenUnconnected=off
  wires:
  In1/1 -> Out1/1

== system eVTOL_Small_nonandlin_algorithm_validation/PID—AttHighControlLaw PID控制器/小于180 ==
  In1 : Inport
  Action Port : ActionPort  ActionPortLabel=else
  Out1 : Outport  VectorParamsAs1DForOutWhenUnconnected=off
  wires:
  In1/1 -> Out1/1

== system eVTOL_Small_nonandlin_algorithm_validation/Subsystem1/Subsystem1 ==
  u : Inport
  y : Inport  Port=2
  ww : Inport  Port=3
  Clock : Clock
  Clock1 : Clock
  Constant : Constant  Value=T
  Constant1 : Constant  Value=g1
  Constant2 : Constant  Value=a_
  Constant3 : Constant  Value=b
  Constant4 : Constant  Value=l1
  Constant5 : Constant  Value=c1_
  Constant6 : Constant  Value=h1
  Constant7 : Constant  Value=ut
  Constant8 : Constant  Value=u_dim
  Constant9 : Constant  Value=x_dim
  Delay : Delay  DelayLength=1  InitialCondition=0
  Delay1 : Delay  DelayLength=1  InitialCondition=0
  Delay2 : Delay  DelayLength=1  InitialCondition=0
  Demux : Demux  Outputs=10
  Demux1 : Demux  Outputs=6
  Demux12 : Demux
  Demux13 : Demux
  Demux2 : Demux  Outputs=6
  MATLAB Function1 : MATLAB Function  TreatAsAtomicUnit=on
  MATLAB Function2 : MATLAB Function  TreatAsAtomicUnit=on
  Mux : Mux
  Mux1 : Mux  Inputs=6
  Mux{2..7,18..21} (10 alike) : Mux  Inputs=2
  Scope1 : Scope  NumInputPorts=6
  Scope14 : Scope  NumInputPorts=4
  Signal Specification : SignalSpecification  Dimensions=[x_dim+u_dim,1]
  Signal Specification1 : SignalSpecification  Dimensions=[u_dim,1]
  Subsystem : Subsystem
  w : Outport
  wires:
  Constant1/1 -> MATLAB Function1/2(g1)
  Constant9/1 -> MATLAB Function2/2(x_dim)
  Constant6/1 -> MATLAB Function1/7(h1)
  MATLAB Function2/1(w_) -> w/1
  u/1 -> Subsystem/1(ut), MATLAB Function1/9(u)
  Constant8/1 -> MATLAB Function2/3(u_dim)
  Delay1/1 -> MATLAB Function1/11(pre_y_)
  Constant5/1 -> MATLAB Function1/6(c1_)
  Constant4/1 -> MATLAB Function1/5(l1)
  Constant3/1 -> MATLAB Function1/4(b)
  Constant/1 -> MATLAB Function1/1(T)
  Subsystem/1(y_) -> Delay1/1, MATLAB Function1/12(y_)
  Constant2/1 -> MATLAB Function1/3(a_)
  y/1 -> Demux1/1, Subsystem/2(y)
  Delay/1 -> MATLAB Function1/8(pre_xx_)
  MATLAB Function1/1(xx_) -> Delay/1, Demux/1, MATLAB Function2/1(xx_)
  MATLAB Function1/2(z) -> Delay2/1
  Clock/1 -> MATLAB Function1/13(t)
  Delay2/1 -> Signal Specification/1
  Signal Specification/1 -> MATLAB Function1/10(pre_z)
  Constant7/1 -> Signal Specification1/1
  Signal Specification1/1 -> MATLAB Function2/4(ut)
  Clock1/1 -> MATLAB Function2/5(t)
  Demux/7 -> Mux/1
  Demux/8 -> Mux/2
  Demux/9 -> Mux/3
  Demux/10 -> Mux/4
  Demux/6 -> Mux1/6
  Demux/1 -> Mux1/1
  Demux/2 -> Mux1/2
  Demux/3 -> Mux1/3
  Demux/4 -> Mux1/4
  Demux/5 -> Mux1/5
  Mux1/1 -> [x_estimate]
  Mux/1 -> [w_estimate]
  Mux21/1 -> Scope14/4  "dr"
  Demux13/2 -> Mux19/2  "de_e"
  Demux12/4 -> Mux21/1  "dr_r"
  Demux12/2 -> Mux19/1  "de_r"
  Demux12/3 -> Mux20/1  "da_r"
  Demux12/1 -> Mux18/1  "dt_r"
  Demux13/1 -> Mux18/2  "dt_e"
  Mux18/1 -> Scope14/1  "dt"
  Demux13/4 -> Mux21/2  "dr_e"
  ww/1 -> Demux12/1
  Demux13/3 -> Mux20/2  "da_e"
  Mux19/1 -> Scope14/2  "de"
  Mux20/1 -> Scope14/3  "da"
  [w_estimate] -> Demux13/1
  Mux6/1 -> Scope1/1  "u"
  Mux7/1 -> Scope1/2  "v"
  Mux2/1 -> Scope1/3  "w"
  Mux3/1 -> Scope1/4  "p"
  Mux4/1 -> Scope1/5  "q"
  Mux5/1 -> Scope1/6  "r"
  Demux1/1 -> Mux6/1
  Demux2/1 -> Mux6/2
  Demux1/2 -> Mux7/1
  Demux2/2 -> Mux7/2
  Demux1/3 -> Mux2/1
  Demux2/3 -> Mux2/2
  Demux1/4 -> Mux3/1
  Demux2/4 -> Mux3/2
  Demux1/5 -> Mux4/1
  Demux2/5 -> Mux4/2
  Demux1/6 -> Mux5/1
  Demux2/6 -> Mux5/2
  [x_estimate] -> Demux2/1
